simulink model "lego_SS_MCC_sim"  (Simulink 10.2)
settings: Solver=ode45  StartTime=0.0  StopTime=10.0  RelTol=1e-3  EnableMultiTasking=on
settings Model: Creator=jacques  LastModifiedBy=etudiant
settings DataIOCC: LimitDataPoints=on
settings OptimizationCC: ExpressionDepthLimit=2147483647
settings DebuggingCC: SolverPrmCheckMsg=warning  StateNameClashWarn=warning

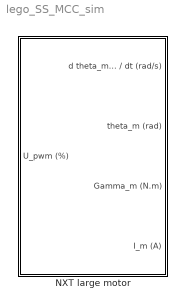
== system lego_SS_MCC_sim ==
  NXT large motor : Subsystem

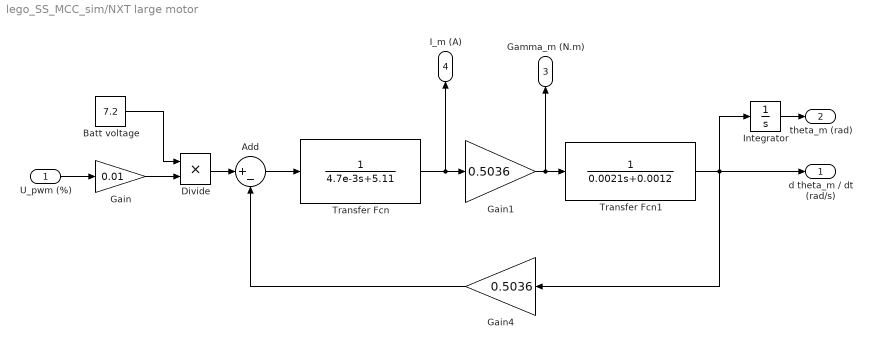
== system lego_SS_MCC_sim/NXT large motor ==
  U_pwm (%) : Inport
  Add : Sum  Inputs=|+-
  Batt voltage : Constant  Value=7.2
  Divide : Product  Inputs=**
  Gain : Gain  Gain=0.01
  Gain1 : Gain  Gain=0.5036
  Gain4 : Gain  Gain=0.5036
  Integrator : Integrator
  Transfer Fcn : TransferFcn  Denominator=[4.7e-3 5.11]
  Transfer Fcn1 : TransferFcn  Denominator=[0.0021 0.0012]
  d theta_m / dt (rad/s) : Outport
  theta_m (rad) : Outport  Port=2
  Gamma_m (N.m) : Outport  Port=3
  I_m (A) : Outport  Port=4
  wires:
  Batt voltage/1 -> Divide/1
  Gain/1 -> Divide/2
  Divide/1 -> Add/1
  Add/1 -> Transfer Fcn/1
  Transfer Fcn/1 -> Gain1/1, I_m (A)/1
  Gain1/1 -> Transfer Fcn1/1, Gamma_m (N.m)/1
  Transfer Fcn1/1 -> Integrator/1, Gain4/1, d theta_m / dt (rad/s)/1
  Gain4/1 -> Add/2
  U_pwm (%)/1 -> Gain/1
  Integrator/1 -> theta_m (rad)/1
